simulink model "TST_EISGov_SelectParameter"  (R2016b)
settings: Solver=FixedStepDiscrete  StartTime=0.0  StopTime=simTime  FixedStep=sampleTime  RelTol=1e-3
values from neighbouring files (symbols this model uses):
  testCase = 1    [initTST_EISGov_SelectParameter_001.m]
libraries: simulink x26, UnitTest_Lib x24
(part 3 of 3)

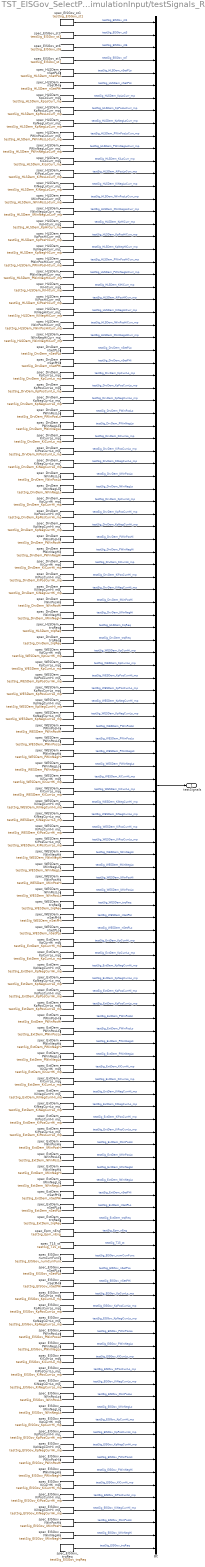
== system TST_EISGov_SelectParameter/simulationInput/testSignals_R001 ==
  BC : BusCreator  Inputs=122
  spec_DrvDem_IWinNegHi : FromWorkspace  VariableName=testSig_DrvDem_IWinNegHi  Interpolate=off  OutputAfterFinalValue=Holding final value
  spec_DrvDem_IWinNegLo : FromWorkspace  VariableName=testSig_DrvDem_IWinNegLo  Interpolate=off  OutputAfterFinalValue=Holding final value
  spec_DrvDem_IWinPosHi : FromWorkspace  VariableName=testSig_DrvDem_IWinPosHi  Interpolate=off  OutputAfterFinalValue=Holding final value
  spec_DrvDem_IWinPosLo : FromWorkspace  VariableName=testSig_DrvDem_IWinPosLo  Interpolate=off  OutputAfterFinalValue=Holding final value
  spec_DrvDem_KiCurrHi_mp : FromWorkspace  VariableName=testSig_DrvDem_KiCurrHi_mp  Interpolate=off  OutputAfterFinalValue=Holding final value
  spec_DrvDem_KiCurrLo_mp : FromWorkspace  VariableName=testSig_DrvDem_KiCurrLo_mp  Interpolate=off  OutputAfterFinalValue=Holding final value
  spec_DrvDem_KiNegCurrHi_mp : FromWorkspace  VariableName=testSig_DrvDem_KiNegCurrHi_mp  Interpolate=off  OutputAfterFinalValue=Holding final value
  spec_DrvDem_KiNegCurrLo_mp : FromWorkspace  VariableName=testSig_DrvDem_KiNegCurrLo_mp  Interpolate=off  OutputAfterFinalValue=Holding final value
  spec_DrvDem_KiPosCurrHi_mp : FromWorkspace  VariableName=testSig_DrvDem_KiPosCurrHi_mp  Interpolate=off  OutputAfterFinalValue=Holding final value
  spec_DrvDem_KiPosCurrLo_mp : FromWorkspace  VariableName=testSig_DrvDem_KiPosCurrLo_mp  Interpolate=off  OutputAfterFinalValue=Holding final value
  spec_DrvDem_KpCurrHi_mp : FromWorkspace  VariableName=testSig_DrvDem_KpCurrHi_mp  Interpolate=off  OutputAfterFinalValue=Holding final value
  spec_DrvDem_KpCurrLo_mp : FromWorkspace  VariableName=testSig_DrvDem_KpCurrLo_mp  Interpolate=off  OutputAfterFinalValue=Holding final value
  spec_DrvDem_KpNegCurrHi_mp : FromWorkspace  VariableName=testSig_DrvDem_KpNegCurrHi_mp  Interpolate=off  OutputAfterFinalValue=Holding final value
  spec_DrvDem_KpNegCurrLo_mp : FromWorkspace  VariableName=testSig_DrvDem_KpNegCurrLo_mp  Interpolate=off  OutputAfterFinalValue=Holding final value
  spec_DrvDem_KpPosCurrHi_mp : FromWorkspace  VariableName=testSig_DrvDem_KpPosCurrHi_mp  Interpolate=off  OutputAfterFinalValue=Holding final value
  spec_DrvDem_KpPosCurrLo_mp : FromWorkspace  VariableName=testSig_DrvDem_KpPosCurrLo_mp  Interpolate=off  OutputAfterFinalValue=Holding final value
  spec_DrvDem_PWinNegHi : FromWorkspace  VariableName=testSig_DrvDem_PWinNegHi  Interpolate=off  OutputAfterFinalValue=Holding final value
  spec_DrvDem_PWinNegLo : FromWorkspace  VariableName=testSig_DrvDem_PWinNegLo  Interpolate=off  OutputAfterFinalValue=Holding final value
  spec_DrvDem_PWinPosHi : FromWorkspace  VariableName=testSig_DrvDem_PWinPosHi  Interpolate=off  OutputAfterFinalValue=Holding final value
  spec_DrvDem_PWinPosLo : FromWorkspace  VariableName=testSig_DrvDem_PWinPosLo  Interpolate=off  OutputAfterFinalValue=Holding final value
  spec_DrvDem_nSetPHi : FromWorkspace  VariableName=testSig_DrvDem_nSetPHi  Interpolate=off  OutputAfterFinalValue=Holding final value
  spec_DrvDem_nSetPLo : FromWorkspace  VariableName=testSig_DrvDem_nSetPLo  Interpolate=off  OutputAfterFinalValue=Holding final value
  spec_DrvDem_trqReq : FromWorkspace  VariableName=testSig_DrvDem_trqReq  Interpolate=off  OutputAfterFinalValue=Holding final value
  spec_EISGov_IWinNegHi : FromWorkspace  VariableName=testSig_EISGov_IWinNegHi  Interpolate=off  OutputAfterFinalValue=Holding final value
  spec_EISGov_IWinNegLo : FromWorkspace  VariableName=testSig_EISGov_IWinNegLo  Interpolate=off  OutputAfterFinalValue=Holding final value
  spec_EISGov_IWinPosHi : FromWorkspace  VariableName=testSig_EISGov_IWinPosHi  Interpolate=off  OutputAfterFinalValue=Holding final value
  spec_EISGov_IWinPosLo : FromWorkspace  VariableName=testSig_EISGov_IWinPosLo  Interpolate=off  OutputAfterFinalValue=Holding final value
  spec_EISGov_KiCurrHi_mp : FromWorkspace  VariableName=testSig_EISGov_KiCurrHi_mp  Interpolate=off  OutputAfterFinalValue=Holding final value
  spec_EISGov_KiCurrLo_mp : FromWorkspace  VariableName=testSig_EISGov_KiCurrLo_mp  Interpolate=off  OutputAfterFinalValue=Holding final value
  spec_EISGov_KiNegCurrHi_mp : FromWorkspace  VariableName=testSig_EISGov_KiNegCurrHi_mp  Interpolate=off  OutputAfterFinalValue=Holding final value
  spec_EISGov_KiNegCurrLo_mp : FromWorkspace  VariableName=testSig_EISGov_KiNegCurrLo_mp  Interpolate=off  OutputAfterFinalValue=Holding final value
  spec_EISGov_KiPosCurrHi_mp : FromWorkspace  VariableName=testSig_EISGov_KiPosCurrHi_mp  Interpolate=off  OutputAfterFinalValue=Holding final value
  spec_EISGov_KiPosCurrLo_mp : FromWorkspace  VariableName=testSig_EISGov_KiPosCurrLo_mp  Interpolate=off  OutputAfterFinalValue=Holding final value
  spec_EISGov_KpCurrHi_mp : FromWorkspace  VariableName=testSig_EISGov_KpCurrHi_mp  Interpolate=off  OutputAfterFinalValue=Holding final value
  spec_EISGov_KpCurrLo_mp : FromWorkspace  VariableName=testSig_EISGov_KpCurrLo_mp  Interpolate=off  OutputAfterFinalValue=Holding final value
  spec_EISGov_KpNegCurrHi_mp : FromWorkspace  VariableName=testSig_EISGov_KpNegCurrHi_mp  Interpolate=off  OutputAfterFinalValue=Holding final value
  spec_EISGov_KpNegCurrLo_mp : FromWorkspace  VariableName=testSig_EISGov_KpNegCurrLo_mp  Interpolate=off  OutputAfterFinalValue=Holding final value
  spec_EISGov_KpPosCurrHi_mp : FromWorkspace  VariableName=testSig_EISGov_KpPosCurrHi_mp  Interpolate=off  OutputAfterFinalValue=Holding final value
  spec_EISGov_KpPosCurrLo_mp : FromWorkspace  VariableName=testSig_EISGov_KpPosCurrLo_mp  Interpolate=off  OutputAfterFinalValue=Holding final value
  spec_EISGov_PWinNegHi : FromWorkspace  VariableName=testSig_EISGov_PWinNegHi  Interpolate=off  OutputAfterFinalValue=Holding final value
  spec_EISGov_PWinNegLo : FromWorkspace  VariableName=testSig_EISGov_PWinNegLo  Interpolate=off  OutputAfterFinalValue=Holding final value
  spec_EISGov_PWinPosHi : FromWorkspace  VariableName=testSig_EISGov_PWinPosHi  Interpolate=off  OutputAfterFinalValue=Holding final value
  spec_EISGov_PWinPosLo : FromWorkspace  VariableName=testSig_EISGov_PWinPosLo  Interpolate=off  OutputAfterFinalValue=Holding final value
  spec_EISGov_nSetPHi : FromWorkspace  VariableName=testSig_EISGov_nSetPHi  Interpolate=off  OutputAfterFinalValue=Holding final value
  spec_EISGov_nSetPLo : FromWorkspace  VariableName=testSig_EISGov_nSetPLo  Interpolate=off  OutputAfterFinalValue=Holding final value
  spec_EISGov_numCurrFunc : FromWorkspace  VariableName=testSig_EISGov_numCurrFunc  Interpolate=off  OutputAfterFinalValue=Holding final value
  spec_EISGov_st1 : FromWorkspace  VariableName=testSig_EISGov_st1  Interpolate=off  OutputAfterFinalValue=Holding final value
  spec_EISGov_st3 : FromWorkspace  VariableName=testSig_EISGov_st3  Interpolate=off  OutputAfterFinalValue=Holding final value
  spec_EISGov_st6 : FromWorkspace  VariableName=testSig_EISGov_st6  Interpolate=off  OutputAfterFinalValue=Holding final value
  spec_EISGov_st7 : FromWorkspace  VariableName=testSig_EISGov_st7  Interpolate=off  OutputAfterFinalValue=Holding final value
  spec_EISGov_trqReq : FromWorkspace  VariableName=testSig_EISGov_trqReq  Interpolate=off  OutputAfterFinalValue=Holding final value
  spec_Epm_nEng : FromWorkspace  VariableName=testSig_Epm_nEng  Interpolate=off  OutputAfterFinalValue=Holding final value
  spec_ExtDem_IWinNegHi : FromWorkspace  VariableName=testSig_ExtDem_IWinNegHi  Interpolate=off  OutputAfterFinalValue=Holding final value
  spec_ExtDem_IWinNegLo : FromWorkspace  VariableName=testSig_ExtDem_IWinNegLo  Interpolate=off  OutputAfterFinalValue=Holding final value
  spec_ExtDem_IWinPosHi : FromWorkspace  VariableName=testSig_ExtDem_IWinPosHi  Interpolate=off  OutputAfterFinalValue=Holding final value
  spec_ExtDem_IWinPosLo : FromWorkspace  VariableName=testSig_ExtDem_IWinPosLo  Interpolate=off  OutputAfterFinalValue=Holding final value
  spec_ExtDem_KiCurrHi_mp : FromWorkspace  VariableName=testSig_ExtDem_KiCurrHi_mp  Interpolate=off  OutputAfterFinalValue=Holding final value
  spec_ExtDem_KiCurrLo_mp : FromWorkspace  VariableName=testSig_ExtDem_KiCurrLo_mp  Interpolate=off  OutputAfterFinalValue=Holding final value
  spec_ExtDem_KiNegCurrHi_mp : FromWorkspace  VariableName=testSig_ExtDem_KiNegCurrHi_mp  Interpolate=off  OutputAfterFinalValue=Holding final value
  spec_ExtDem_KiNegCurrLo_mp : FromWorkspace  VariableName=testSig_ExtDem_KiNegCurrLo_mp  Interpolate=off  OutputAfterFinalValue=Holding final value
  spec_ExtDem_KiPosCurrHi_mp : FromWorkspace  VariableName=testSig_ExtDem_KiPosCurrHi_mp  Interpolate=off  OutputAfterFinalValue=Holding final value
  spec_ExtDem_KiPosCurrLo_mp : FromWorkspace  VariableName=testSig_ExtDem_KiPosCurrLo_mp  Interpolate=off  OutputAfterFinalValue=Holding final value
  spec_ExtDem_KpCurrHi_mp : FromWorkspace  VariableName=testSig_ExtDem_KpCurrHi_mp  Interpolate=off  OutputAfterFinalValue=Holding final value
  spec_ExtDem_KpCurrLo_mp : FromWorkspace  VariableName=testSig_ExtDem_KpCurrLo_mp  Interpolate=off  OutputAfterFinalValue=Holding final value
  spec_ExtDem_KpNegCurrHi_mp : FromWorkspace  VariableName=testSig_ExtDem_KpNegCurrHi_mp  Interpolate=off  OutputAfterFinalValue=Holding final value
  spec_ExtDem_KpNegCurrLo_mp : FromWorkspace  VariableName=testSig_ExtDem_KpNegCurrLo_mp  Interpolate=off  OutputAfterFinalValue=Holding final value
  spec_ExtDem_KpPosCurrHi_mp : FromWorkspace  VariableName=testSig_ExtDem_KpPosCurrHi_mp  Interpolate=off  OutputAfterFinalValue=Holding final value
  spec_ExtDem_KpPosCurrLo_mp : FromWorkspace  VariableName=testSig_ExtDem_KpPosCurrLo_mp  Interpolate=off  OutputAfterFinalValue=Holding final value
  spec_ExtDem_PWinNegHi : FromWorkspace  VariableName=testSig_ExtDem_PWinNegHi  Interpolate=off  OutputAfterFinalValue=Holding final value
  spec_ExtDem_PWinNegLo : FromWorkspace  VariableName=testSig_ExtDem_PWinNegLo  Interpolate=off  OutputAfterFinalValue=Holding final value
  spec_ExtDem_PWinPosHi : FromWorkspace  VariableName=testSig_ExtDem_PWinPosHi  Interpolate=off  OutputAfterFinalValue=Holding final value
  spec_ExtDem_PWinPosLo : FromWorkspace  VariableName=testSig_ExtDem_PWinPosLo  Interpolate=off  OutputAfterFinalValue=Holding final value
  spec_ExtDem_nSetPHi : FromWorkspace  VariableName=testSig_ExtDem_nSetPHi  Interpolate=off  OutputAfterFinalValue=Holding final value
  spec_ExtDem_nSetPLo : FromWorkspace  VariableName=testSig_ExtDem_nSetPLo  Interpolate=off  OutputAfterFinalValue=Holding final value
  spec_ExtDem_trqReq : FromWorkspace  VariableName=testSig_ExtDem_trqReq  Interpolate=off  OutputAfterFinalValue=Holding final value
  spec_HLSDem_IWinNegHiCurr_mp : FromWorkspace  VariableName=testSig_HLSDem_IWinNegHiCurr_mp  Interpolate=off  OutputAfterFinalValue=Holding final value
  spec_HLSDem_IWinNegLoCurr_mp : FromWorkspace  VariableName=testSig_HLSDem_IWinNegLoCurr_mp  Interpolate=off  OutputAfterFinalValue=Holding final value
  spec_HLSDem_IWinPosHiCurr_mp : FromWorkspace  VariableName=testSig_HLSDem_IWinPosHiCurr_mp  Interpolate=off  OutputAfterFinalValue=Holding final value
  spec_HLSDem_IWinPosLoCurr_mp : FromWorkspace  VariableName=testSig_HLSDem_IWinPosLoCurr_mp  Interpolate=off  OutputAfterFinalValue=Holding final value
  spec_HLSDem_KiHiCurr_mp : FromWorkspace  VariableName=testSig_HLSDem_KiHiCurr_mp  Interpolate=off  OutputAfterFinalValue=Holding final value
  spec_HLSDem_KiLoCurr_mp : FromWorkspace  VariableName=testSig_HLSDem_KiLoCurr_mp  Interpolate=off  OutputAfterFinalValue=Holding final value
  spec_HLSDem_KiNegHiCurr_mp : FromWorkspace  VariableName=testSig_HLSDem_KiNegHiCurr_mp  Interpolate=off  OutputAfterFinalValue=Holding final value
  spec_HLSDem_KiNegLoCurr_mp : FromWorkspace  VariableName=testSig_HLSDem_KiNegLoCurr_mp  Interpolate=off  OutputAfterFinalValue=Holding final value
  spec_HLSDem_KiPosHiCurr_mp : FromWorkspace  VariableName=testSig_HLSDem_KiPosHiCurr_mp  Interpolate=off  OutputAfterFinalValue=Holding final value
  spec_HLSDem_KiPosLoCurr_mp : FromWorkspace  VariableName=testSig_HLSDem_KiPosLoCurr_mp  Interpolate=off  OutputAfterFinalValue=Holding final value
  spec_HLSDem_KpHiCurr_mp : FromWorkspace  VariableName=testSig_HLSDem_KpHiCurr_mp  Interpolate=off  OutputAfterFinalValue=Holding final value
  spec_HLSDem_KpLoCurr_mp : FromWorkspace  VariableName=testSig_HLSDem_KpLoCurr_mp  Interpolate=off  OutputAfterFinalValue=Holding final value
  spec_HLSDem_KpNegHiCurr_mp : FromWorkspace  VariableName=testSig_HLSDem_KpNegHiCurr_mp  Interpolate=off  OutputAfterFinalValue=Holding final value
  spec_HLSDem_KpNegLoCurr_mp : FromWorkspace  VariableName=testSig_HLSDem_KpNegLoCurr_mp  Interpolate=off  OutputAfterFinalValue=Holding final value
  spec_HLSDem_KpPosHiCurr_mp : FromWorkspace  VariableName=testSig_HLSDem_KpPosHiCurr_mp  Interpolate=off  OutputAfterFinalValue=Holding final value
  spec_HLSDem_KpPosLoCurr_mp : FromWorkspace  VariableName=testSig_HLSDem_KpPosLoCurr_mp  Interpolate=off  OutputAfterFinalValue=Holding final value
  spec_HLSDem_PWinNegHiCurr_mp : FromWorkspace  VariableName=testSig_HLSDem_PWinNegHiCurr_mp  Interpolate=off  OutputAfterFinalValue=Holding final value
  spec_HLSDem_PWinNegLoCurr_mp : FromWorkspace  VariableName=testSig_HLSDem_PWinNegLoCurr_mp  Interpolate=off  OutputAfterFinalValue=Holding final value
  spec_HLSDem_PWinPosHiCurr_mp : FromWorkspace  VariableName=testSig_HLSDem_PWinPosHiCurr_mp  Interpolate=off  OutputAfterFinalValue=Holding final value
  spec_HLSDem_PWinPosLoCurr_mp : FromWorkspace  VariableName=testSig_HLSDem_PWinPosLoCurr_mp  Interpolate=off  OutputAfterFinalValue=Holding final value
  spec_HLSDem_nSetPHi : FromWorkspace  VariableName=testSig_HLSDem_nSetPHi  Interpolate=off  OutputAfterFinalValue=Holding final value
  spec_HLSDem_nSetPLo : FromWorkspace  VariableName=testSig_HLSDem_nSetPLo  Interpolate=off  OutputAfterFinalValue=Holding final value
  spec_HLSDem_trqReq : FromWorkspace  VariableName=testSig_HLSDem_trqReq  Interpolate=off  OutputAfterFinalValue=Holding final value
  spec_T15_st : FromWorkspace  VariableName=testSig_T15_st  Interpolate=off  OutputAfterFinalValue=Holding final value
  spec_WESDem_IWinNegHi : FromWorkspace  VariableName=testSig_WESDem_IWinNegHi  Interpolate=off  OutputAfterFinalValue=Holding final value
  spec_WESDem_IWinNegLo : FromWorkspace  VariableName=testSig_WESDem_IWinNegLo  Interpolate=off  OutputAfterFinalValue=Holding final value
  spec_WESDem_IWinPosHi : FromWorkspace  VariableName=testSig_WESDem_IWinPosHi  Interpolate=off  OutputAfterFinalValue=Holding final value
  spec_WESDem_IWinPosLo : FromWorkspace  VariableName=testSig_WESDem_IWinPosLo  Interpolate=off  OutputAfterFinalValue=Holding final value
  spec_WESDem_KiCurrHi_mp : FromWorkspace  VariableName=testSig_WESDem_KiCurrHi_mp  Interpolate=off  OutputAfterFinalValue=Holding final value
  spec_WESDem_KiCurrLo_mp : FromWorkspace  VariableName=testSig_WESDem_KiCurrLo_mp  Interpolate=off  OutputAfterFinalValue=Holding final value
  spec_WESDem_KiNegCurrHi_mp : FromWorkspace  VariableName=testSig_WESDem_KiNegCurrHi_mp  Interpolate=off  OutputAfterFinalValue=Holding final value
  spec_WESDem_KiNegCurrLo_mp : FromWorkspace  VariableName=testSig_WESDem_KiNegCurrLo_mp  Interpolate=off  OutputAfterFinalValue=Holding final value
  spec_WESDem_KiPosCurrHi_mp : FromWorkspace  VariableName=testSig_WESDem_KiPosCurrHi_mp  Interpolate=off  OutputAfterFinalValue=Holding final value
  spec_WESDem_KiPosCurrLo_mp : FromWorkspace  VariableName=testSig_WESDem_KiPosCurrLo_mp  Interpolate=off  OutputAfterFinalValue=Holding final value
  spec_WESDem_KpCurrHi_mp : FromWorkspace  VariableName=testSig_WESDem_KpCurrHi_mp  Interpolate=off  OutputAfterFinalValue=Holding final value
  spec_WESDem_KpCurrLo_mp : FromWorkspace  VariableName=testSig_WESDem_KpCurrLo_mp  Interpolate=off  OutputAfterFinalValue=Holding final value
  spec_WESDem_KpNegCurrHi_mp : FromWorkspace  VariableName=testSig_WESDem_KpNegCurrHi_mp  Interpolate=off  OutputAfterFinalValue=Holding final value
  spec_WESDem_KpNegCurrLo_mp : FromWorkspace  VariableName=testSig_WESDem_KpNegCurrLo_mp  Interpolate=off  OutputAfterFinalValue=Holding final value
  spec_WESDem_KpPosCurrHi_mp : FromWorkspace  VariableName=testSig_WESDem_KpPosCurrHi_mp  Interpolate=off  OutputAfterFinalValue=Holding final value
  spec_WESDem_KpPosCurrLo_mp : FromWorkspace  VariableName=testSig_WESDem_KpPosCurrLo_mp  Interpolate=off  OutputAfterFinalValue=Holding final value
  spec_WESDem_PWinNegHi : FromWorkspace  VariableName=testSig_WESDem_PWinNegHi  Interpolate=off  OutputAfterFinalValue=Holding final value
  spec_WESDem_PWinNegLo : FromWorkspace  VariableName=testSig_WESDem_PWinNegLo  Interpolate=off  OutputAfterFinalValue=Holding final value
  spec_WESDem_PWinPosHi : FromWorkspace  VariableName=testSig_WESDem_PWinPosHi  Interpolate=off  OutputAfterFinalValue=Holding final value
  spec_WESDem_PWinPosLo : FromWorkspace  VariableName=testSig_WESDem_PWinPosLo  Interpolate=off  OutputAfterFinalValue=Holding final value
  spec_WESDem_nSetPHi : FromWorkspace  VariableName=testSig_WESDem_nSetPHi  Interpolate=off  OutputAfterFinalValue=Holding final value
  spec_WESDem_nSetPLo : FromWorkspace  VariableName=testSig_WESDem_nSetPLo  Interpolate=off  OutputAfterFinalValue=Holding final value
  spec_WESDem_trqReq : FromWorkspace  VariableName=testSig_WESDem_trqReq  Interpolate=off  OutputAfterFinalValue=Holding final value
  testSignals : Outport
  wires:
  BC/1 -> testSignals/1
  spec_EISGov_st1/1 -> BC/1  "testSig_EISGov_st1"
  spec_EISGov_st3/1 -> BC/2  "testSig_EISGov_st3"
  spec_EISGov_st6/1 -> BC/3  "testSig_EISGov_st6"
  spec_EISGov_st7/1 -> BC/4  "testSig_EISGov_st7"
  spec_HLSDem_nSetPLo/1 -> BC/5  "testSig_HLSDem_nSetPLo"
  spec_HLSDem_nSetPHi/1 -> BC/6  "testSig_HLSDem_nSetPHi"
  spec_HLSDem_KpLoCurr_mp/1 -> BC/7  "testSig_HLSDem_KpLoCurr_mp"
  spec_HLSDem_KpPosLoCurr_mp/1 -> BC/8  "testSig_HLSDem_KpPosLoCurr_mp"
  spec_HLSDem_KpNegLoCurr_mp/1 -> BC/9  "testSig_HLSDem_KpNegLoCurr_mp"
  spec_HLSDem_PWinPosLoCurr_mp/1 -> BC/10  "testSig_HLSDem_PWinPosLoCurr_mp"
  spec_HLSDem_PWinNegLoCurr_mp/1 -> BC/11  "testSig_HLSDem_PWinNegLoCurr_mp"
  spec_HLSDem_KiLoCurr_mp/1 -> BC/12  "testSig_HLSDem_KiLoCurr_mp"
  spec_HLSDem_KiPosLoCurr_mp/1 -> BC/13  "testSig_HLSDem_KiPosLoCurr_mp"
  spec_HLSDem_KiNegLoCurr_mp/1 -> BC/14  "testSig_HLSDem_KiNegLoCurr_mp"
  spec_HLSDem_IWinPosLoCurr_mp/1 -> BC/15  "testSig_HLSDem_IWinPosLoCurr_mp"
  spec_HLSDem_IWinNegLoCurr_mp/1 -> BC/16  "testSig_HLSDem_IWinNegLoCurr_mp"
  spec_HLSDem_KpHiCurr_mp/1 -> BC/17  "testSig_HLSDem_KpHiCurr_mp"
  spec_HLSDem_KpPosHiCurr_mp/1 -> BC/18  "testSig_HLSDem_KpPosHiCurr_mp"
  spec_HLSDem_KpNegHiCurr_mp/1 -> BC/19  "testSig_HLSDem_KpNegHiCurr_mp"
  spec_HLSDem_PWinPosHiCurr_mp/1 -> BC/20  "testSig_HLSDem_PWinPosHiCurr_mp"
  spec_HLSDem_PWinNegHiCurr_mp/1 -> BC/21  "testSig_HLSDem_PWinNegHiCurr_mp"
  spec_HLSDem_KiHiCurr_mp/1 -> BC/22  "testSig_HLSDem_KiHiCurr_mp"
  spec_HLSDem_KiPosHiCurr_mp/1 -> BC/23  "testSig_HLSDem_KiPosHiCurr_mp"
  spec_HLSDem_KiNegHiCurr_mp/1 -> BC/24  "testSig_HLSDem_KiNegHiCurr_mp"
  spec_HLSDem_IWinPosHiCurr_mp/1 -> BC/25  "testSig_HLSDem_IWinPosHiCurr_mp"
  spec_HLSDem_IWinNegHiCurr_mp/1 -> BC/26  "testSig_HLSDem_IWinNegHiCurr_mp"
  spec_DrvDem_nSetPLo/1 -> BC/27  "testSig_DrvDem_nSetPLo"
  spec_DrvDem_nSetPHi/1 -> BC/28  "testSig_DrvDem_nSetPHi"
  spec_DrvDem_KpCurrLo_mp/1 -> BC/29  "testSig_DrvDem_KpCurrLo_mp"
  spec_DrvDem_KpPosCurrLo_mp/1 -> BC/30  "testSig_DrvDem_KpPosCurrLo_mp"
  spec_DrvDem_KpNegCurrLo_mp/1 -> BC/31  "testSig_DrvDem_KpNegCurrLo_mp"
  spec_DrvDem_PWinPosLo/1 -> BC/32  "testSig_DrvDem_PWinPosLo"
  spec_DrvDem_PWinNegLo/1 -> BC/33  "testSig_DrvDem_PWinNegLo"
  spec_DrvDem_KiCurrLo_mp/1 -> BC/34  "testSig_DrvDem_KiCurrLo_mp"
  spec_DrvDem_KiPosCurrLo_mp/1 -> BC/35  "testSig_DrvDem_KiPosCurrLo_mp"
  spec_DrvDem_KiNegCurrLo_mp/1 -> BC/36  "testSig_DrvDem_KiNegCurrLo_mp"
  spec_DrvDem_IWinPosLo/1 -> BC/37  "testSig_DrvDem_IWinPosLo"
  spec_DrvDem_IWinNegLo/1 -> BC/38  "testSig_DrvDem_IWinNegLo"
  spec_DrvDem_KpCurrHi_mp/1 -> BC/39  "testSig_DrvDem_KpCurrHi_mp"
  spec_DrvDem_KpPosCurrHi_mp/1 -> BC/40  "testSig_DrvDem_KpPosCurrHi_mp"
  spec_DrvDem_KpNegCurrHi_mp/1 -> BC/41  "testSig_DrvDem_KpNegCurrHi_mp"
  spec_DrvDem_PWinPosHi/1 -> BC/42  "testSig_DrvDem_PWinPosHi"
  spec_DrvDem_PWinNegHi/1 -> BC/43  "testSig_DrvDem_PWinNegHi"
  spec_DrvDem_KiCurrHi_mp/1 -> BC/44  "testSig_DrvDem_KiCurrHi_mp"
  spec_DrvDem_KiPosCurrHi_mp/1 -> BC/45  "testSig_DrvDem_KiPosCurrHi_mp"
  spec_DrvDem_KiNegCurrHi_mp/1 -> BC/46  "testSig_DrvDem_KiNegCurrHi_mp"
  spec_DrvDem_IWinPosHi/1 -> BC/47  "testSig_DrvDem_IWinPosHi"
  spec_DrvDem_IWinNegHi/1 -> BC/48  "testSig_DrvDem_IWinNegHi"
  spec_HLSDem_trqReq/1 -> BC/49  "testSig_HLSDem_trqReq"
  spec_DrvDem_trqReq/1 -> BC/50  "testSig_DrvDem_trqReq"
  spec_WESDem_KpCurrHi_mp/1 -> BC/51  "testSig_WESDem_KpCurrHi_mp"
  spec_WESDem_KpCurrLo_mp/1 -> BC/52  "testSig_WESDem_KpCurrLo_mp"
  spec_WESDem_KpPosCurrHi_mp/1 -> BC/53  "testSig_WESDem_KpPosCurrHi_mp"
  spec_WESDem_KpPosCurrLo_mp/1 -> BC/54  "testSig_WESDem_KpPosCurrLo_mp"
  spec_WESDem_KpNegCurrHi_mp/1 -> BC/55  "testSig_WESDem_KpNegCurrHi_mp"
  spec_WESDem_KpNegCurrLo_mp/1 -> BC/56  "testSig_WESDem_KpNegCurrLo_mp"
  spec_WESDem_PWinPosHi/1 -> BC/57  "testSig_WESDem_PWinPosHi"
  spec_WESDem_PWinPosLo/1 -> BC/58  "testSig_WESDem_PWinPosLo"
  spec_WESDem_PWinNegHi/1 -> BC/59  "testSig_WESDem_PWinNegHi"
  spec_WESDem_PWinNegLo/1 -> BC/60  "testSig_WESDem_PWinNegLo"
  spec_WESDem_KiCurrHi_mp/1 -> BC/61  "testSig_WESDem_KiCurrHi_mp"
  spec_WESDem_KiCurrLo_mp/1 -> BC/62  "testSig_WESDem_KiCurrLo_mp"
  spec_WESDem_KiNegCurrHi_mp/1 -> BC/63  "testSig_WESDem_KiNegCurrHi_mp"
  spec_WESDem_KiNegCurrLo_mp/1 -> BC/64  "testSig_WESDem_KiNegCurrLo_mp"
  spec_WESDem_KiPosCurrHi_mp/1 -> BC/65  "testSig_WESDem_KiPosCurrHi_mp"
  spec_WESDem_KiPosCurrLo_mp/1 -> BC/66  "testSig_WESDem_KiPosCurrLo_mp"
  spec_WESDem_IWinNegHi/1 -> BC/67  "testSig_WESDem_IWinNegHi"
  spec_WESDem_IWinNegLo/1 -> BC/68  "testSig_WESDem_IWinNegLo"
  spec_WESDem_IWinPosHi/1 -> BC/69  "testSig_WESDem_IWinPosHi"
  spec_WESDem_IWinPosLo/1 -> BC/70  "testSig_WESDem_IWinPosLo"
  spec_WESDem_trqReq/1 -> BC/71  "testSig_WESDem_trqReq"
  spec_WESDem_nSetPHi/1 -> BC/72  "testSig_WESDem_nSetPHi"
  spec_WESDem_nSetPLo/1 -> BC/73  "testSig_WESDem_nSetPLo"
  spec_ExtDem_KpCurrHi_mp/1 -> BC/74  "testSig_ExtDem_KpCurrHi_mp"
  spec_ExtDem_KpCurrLo_mp/1 -> BC/75  "testSig_ExtDem_KpCurrLo_mp"
  spec_ExtDem_KpNegCurrHi_mp/1 -> BC/76  "testSig_ExtDem_KpNegCurrHi_mp"
  spec_ExtDem_KpNegCurrLo_mp/1 -> BC/77  "testSig_ExtDem_KpNegCurrLo_mp"
  spec_ExtDem_KpPosCurrHi_mp/1 -> BC/78  "testSig_ExtDem_KpPosCurrHi_mp"
  spec_ExtDem_KpPosCurrLo_mp/1 -> BC/79  "testSig_ExtDem_KpPosCurrLo_mp"
  spec_ExtDem_PWinPosHi/1 -> BC/80  "testSig_ExtDem_PWinPosHi"
  spec_ExtDem_PWinPosLo/1 -> BC/81  "testSig_ExtDem_PWinPosLo"
  spec_ExtDem_PWinNegHi/1 -> BC/82  "testSig_ExtDem_PWinNegHi"
  spec_ExtDem_PWinNegLo/1 -> BC/83  "testSig_ExtDem_PWinNegLo"
  spec_ExtDem_KiCurrHi_mp/1 -> BC/84  "testSig_ExtDem_KiCurrHi_mp"
  spec_ExtDem_KiCurrLo_mp/1 -> BC/85  "testSig_ExtDem_KiCurrLo_mp"
  spec_ExtDem_KiNegCurrHi_mp/1 -> BC/86  "testSig_ExtDem_KiNegCurrHi_mp"
  spec_ExtDem_KiNegCurrLo_mp/1 -> BC/87  "testSig_ExtDem_KiNegCurrLo_mp"
  spec_ExtDem_KiPosCurrHi_mp/1 -> BC/88  "testSig_ExtDem_KiPosCurrHi_mp"
  spec_ExtDem_KiPosCurrLo_mp/1 -> BC/89  "testSig_ExtDem_KiPosCurrLo_mp"
  spec_ExtDem_IWinPosHi/1 -> BC/90  "testSig_ExtDem_IWinPosHi"
  spec_ExtDem_IWinPosLo/1 -> BC/91  "testSig_ExtDem_IWinPosLo"
  spec_ExtDem_IWinNegHi/1 -> BC/92  "testSig_ExtDem_IWinNegHi"
  spec_ExtDem_IWinNegLo/1 -> BC/93  "testSig_ExtDem_IWinNegLo"
  spec_ExtDem_nSetPHi/1 -> BC/94  "testSig_ExtDem_nSetPHi"
  spec_ExtDem_nSetPLo/1 -> BC/95  "testSig_ExtDem_nSetPLo"
  spec_ExtDem_trqReq/1 -> BC/96  "testSig_ExtDem_trqReq"
  spec_Epm_nEng/1 -> BC/97  "testSig_Epm_nEng"
  spec_T15_st/1 -> BC/98  "testSig_T15_st"
  spec_EISGov_numCurrFunc/1 -> BC/99  "testSig_EISGov_numCurrFunc"
  spec_EISGov_nSetPLo/1 -> BC/100  "testSig_EISGov_nSetPLo"
  spec_EISGov_nSetPHi/1 -> BC/101  "testSig_EISGov_nSetPHi"
  spec_EISGov_KpCurrLo_mp/1 -> BC/102  "testSig_EISGov_KpCurrLo_mp"
  spec_EISGov_KpPosCurrLo_mp/1 -> BC/103  "testSig_EISGov_KpPosCurrLo_mp"
  spec_EISGov_KpNegCurrLo_mp/1 -> BC/104  "testSig_EISGov_KpNegCurrLo_mp"
  spec_EISGov_PWinPosLo/1 -> BC/105  "testSig_EISGov_PWinPosLo"
  spec_EISGov_PWinNegLo/1 -> BC/106  "testSig_EISGov_PWinNegLo"
  spec_EISGov_KiCurrLo_mp/1 -> BC/107  "testSig_EISGov_KiCurrLo_mp"
  spec_EISGov_KiPosCurrLo_mp/1 -> BC/108  "testSig_EISGov_KiPosCurrLo_mp"
  spec_EISGov_KiNegCurrLo_mp/1 -> BC/109  "testSig_EISGov_KiNegCurrLo_mp"
  spec_EISGov_IWinPosLo/1 -> BC/110  "testSig_EISGov_IWinPosLo"
  spec_EISGov_IWinNegLo/1 -> BC/111  "testSig_EISGov_IWinNegLo"
  spec_EISGov_KpCurrHi_mp/1 -> BC/112  "testSig_EISGov_KpCurrHi_mp"
  spec_EISGov_KpPosCurrHi_mp/1 -> BC/113  "testSig_EISGov_KpPosCurrHi_mp"
  spec_EISGov_KpNegCurrHi_mp/1 -> BC/114  "testSig_EISGov_KpNegCurrHi_mp"
  spec_EISGov_PWinPosHi/1 -> BC/115  "testSig_EISGov_PWinPosHi"
  spec_EISGov_PWinNegHi/1 -> BC/116  "testSig_EISGov_PWinNegHi"
  spec_EISGov_KiCurrHi_mp/1 -> BC/117  "testSig_EISGov_KiCurrHi_mp"
  spec_EISGov_KiPosCurrHi_mp/1 -> BC/118  "testSig_EISGov_KiPosCurrHi_mp"
  spec_EISGov_KiNegCurrHi_mp/1 -> BC/119  "testSig_EISGov_KiNegCurrHi_mp"
  spec_EISGov_IWinPosHi/1 -> BC/120  "testSig_EISGov_IWinPosHi"
  spec_EISGov_IWinNegHi/1 -> BC/121  "testSig_EISGov_IWinNegHi"
  spec_EISGov_trqReq/1 -> BC/122  "testSig_EISGov_trqReq"

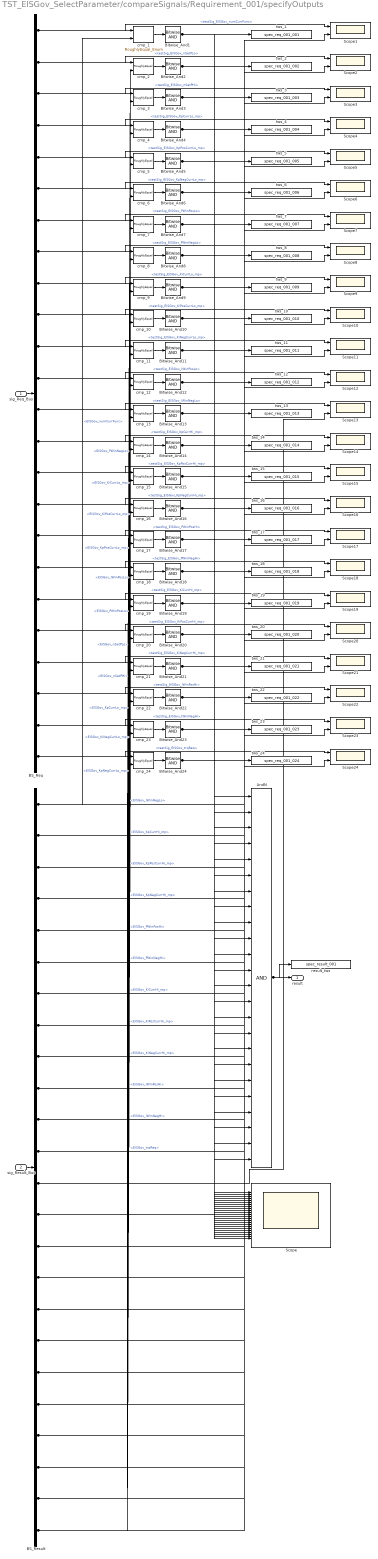
== system TST_EISGov_SelectParameter/compareSignals/Requirement_001/specifyOutputs ==
  sig_Req_Bus : Inport
  sig_Result_Bus : Inport  Port=2
  AndN : Logic  Inputs=24
  BS_Req : BusSelector  OutputSignals=testSig_EISGov_numCurrFunc,testSig_EISGov_nSetPLo,testSig_EISGov_nSetPHi,testSig_EISGov_KpCurrLo_mp,testSig_EISGov_KpPosCurrLo_mp,testSig_EISGov_KpNegCurrLo_mp,testSig_EISGov_PWinPosLo,testSig_EISGov_PWinNegLo,testSig_EISGov_KiCurrLo_mp,testSig_EISGov_KiPosCurrLo_mp,testSig_EISGov_KiNegCurrLo_mp,testSig_EISGov_IWinPosLo,testSig_EISGov_IWinNegLo,testSig_EISGov_KpCurrHi_mp,testSig_EISGov_KpPosCurrHi_mp,testSig_EISGov_KpNegCurrHi_mp,testSig_EISGov_PWinPosHi,testSig_EISGov_PWinNegHi,testSig_EISGov_KiCurrHi_mp,testSig_EISGov_KiPosCurrHi_mp,testSig_EISGov_KiNegCurrHi_mp,testSig_EISGov_IWinPosHi,testSig_EISGov_IWinNegHi,testSig_EISGov_trqReq
  BS_Result : BusSelector  OutputSignals=EISGov_numCurrFunc,EISGov_nSetPLo,EISGov_nSetPHi,EISGov_KpCurrLo_mp,EISGov_KpPosCurrLo_mp,EISGov_KpNegCurrLo_mp,EISGov_PWinPosLo,EISGov_PWinNegLo,EISGov_KiCurrLo_mp,EISGov_KiPosCurrLo_mp,EISGov_KiNegCurrLo_mp,EISGov_IWinPosLo,EISGov_IWinNegLo,EISGov_KpCurrHi_mp,EISGov_KpPosCurrHi_mp,EISGov_KpNegCurrHi_mp,EISGov_PWinPosHi,EISGov_PWinNegHi,EISGov_KiCurrHi_mp,EISGov_KiPosCurrHi_mp,EISGov_KiNegCurrHi_mp,EISGov_IWinPosHi,EISGov_IWinNegHi,EISGov_trqReq
  Bitwise_And{1..24} (24 alike) : simulink/Logic and Bit Operations/Bitwise Operator  logicop=AND  UseBitMask=off  BitMask=bin2dec('11011001')  BitMaskRealWorld=Stored Integer
  Scope : Scope  NumInputPorts=24
  Scope{1..24} (24 alike) : Scope  NumInputPorts=2
  cmp_1 : UnitTest_Lib/RoughlyEqual_Enum  slope=0.1
  cmp_{2..24} (23 alike) : UnitTest_Lib/RoughlyEqual  slope=0.1
  result_tws : ToWorkspace  VariableName=spec_result_001
  tws_1 : ToWorkspace  VariableName=spec_req_001_001
  tws_10 : ToWorkspace  VariableName=spec_req_001_010
  tws_11 : ToWorkspace  VariableName=spec_req_001_011
  tws_12 : ToWorkspace  VariableName=spec_req_001_012
  tws_13 : ToWorkspace  VariableName=spec_req_001_013
  tws_14 : ToWorkspace  VariableName=spec_req_001_014
  tws_15 : ToWorkspace  VariableName=spec_req_001_015
  tws_16 : ToWorkspace  VariableName=spec_req_001_016
  tws_17 : ToWorkspace  VariableName=spec_req_001_017
  tws_18 : ToWorkspace  VariableName=spec_req_001_018
  tws_19 : ToWorkspace  VariableName=spec_req_001_019
  tws_2 : ToWorkspace  VariableName=spec_req_001_002
  tws_20 : ToWorkspace  VariableName=spec_req_001_020
  tws_21 : ToWorkspace  VariableName=spec_req_001_021
  tws_22 : ToWorkspace  VariableName=spec_req_001_022
  tws_23 : ToWorkspace  VariableName=spec_req_001_023
  tws_24 : ToWorkspace  VariableName=spec_req_001_024
  tws_3 : ToWorkspace  VariableName=spec_req_001_003
  tws_4 : ToWorkspace  VariableName=spec_req_001_004
  tws_5 : ToWorkspace  VariableName=spec_req_001_005
  tws_6 : ToWorkspace  VariableName=spec_req_001_006
  tws_7 : ToWorkspace  VariableName=spec_req_001_007
  tws_8 : ToWorkspace  VariableName=spec_req_001_008
  tws_9 : ToWorkspace  VariableName=spec_req_001_009
  result : Outport
  wires:
  sig_Req_Bus/1 -> BS_Req/1
  sig_Result_Bus/1 -> BS_Result/1
  AndN/1 -> result/1, result_tws/1
  BS_Req/1 -> cmp_1/1, Scope1/1  "<testSig_EISGov_numCurrFunc>"
  BS_Result/1 -> cmp_1/2, Scope1/2  "<EISGov_numCurrFunc>"
  cmp_1/1 -> Bitwise_And1/1
  Bitwise_And1/1 -> tws_1/1, AndN/1, Scope/1
  BS_Req/2 -> cmp_2/1, Scope2/1  "<testSig_EISGov_nSetPLo>"
  BS_Result/2 -> cmp_2/2, Scope2/2  "<EISGov_nSetPLo>"
  cmp_2/1 -> Bitwise_And2/1
  Bitwise_And2/1 -> tws_2/1, AndN/2, Scope/2
  BS_Req/3 -> cmp_3/1, Scope3/1  "<testSig_EISGov_nSetPHi>"
  BS_Result/3 -> cmp_3/2, Scope3/2  "<EISGov_nSetPHi>"
  cmp_3/1 -> Bitwise_And3/1
  Bitwise_And3/1 -> tws_3/1, AndN/3, Scope/3
  BS_Req/4 -> cmp_4/1, Scope4/1  "<testSig_EISGov_KpCurrLo_mp>"
  BS_Result/4 -> cmp_4/2, Scope4/2  "<EISGov_KpCurrLo_mp>"
  cmp_4/1 -> Bitwise_And4/1
  Bitwise_And4/1 -> tws_4/1, AndN/4, Scope/4
  BS_Req/5 -> cmp_5/1, Scope5/1  "<testSig_EISGov_KpPosCurrLo_mp>"
  BS_Result/5 -> cmp_5/2, Scope5/2  "<EISGov_KpPosCurrLo_mp>"
  cmp_5/1 -> Bitwise_And5/1
  Bitwise_And5/1 -> tws_5/1, AndN/5, Scope/5
  BS_Req/6 -> cmp_6/1, Scope6/1  "<testSig_EISGov_KpNegCurrLo_mp>"
  BS_Result/6 -> cmp_6/2, Scope6/2  "<EISGov_KpNegCurrLo_mp>"
  cmp_6/1 -> Bitwise_And6/1
  Bitwise_And6/1 -> tws_6/1, AndN/6, Scope/6
  BS_Req/7 -> cmp_7/1, Scope7/1  "<testSig_EISGov_PWinPosLo>"
  BS_Result/7 -> cmp_7/2, Scope7/2  "<EISGov_PWinPosLo>"
  cmp_7/1 -> Bitwise_And7/1
  Bitwise_And7/1 -> tws_7/1, AndN/7, Scope/7
  BS_Req/8 -> cmp_8/1, Scope8/1  "<testSig_EISGov_PWinNegLo>"
  BS_Result/8 -> cmp_8/2, Scope8/2  "<EISGov_PWinNegLo>"
  cmp_8/1 -> Bitwise_And8/1
  Bitwise_And8/1 -> tws_8/1, AndN/8, Scope/8
  BS_Req/9 -> cmp_9/1, Scope9/1  "<testSig_EISGov_KiCurrLo_mp>"
  BS_Result/9 -> cmp_9/2, Scope9/2  "<EISGov_KiCurrLo_mp>"
  cmp_9/1 -> Bitwise_And9/1
  Bitwise_And9/1 -> tws_9/1, AndN/9, Scope/9
  BS_Req/10 -> cmp_10/1, Scope10/1  "<testSig_EISGov_KiPosCurrLo_mp>"
  BS_Result/10 -> cmp_10/2, Scope10/2  "<EISGov_KiPosCurrLo_mp>"
  cmp_10/1 -> Bitwise_And10/1
  Bitwise_And10/1 -> tws_10/1, AndN/10, Scope/10
  BS_Req/11 -> cmp_11/1, Scope11/1  "<testSig_EISGov_KiNegCurrLo_mp>"
  BS_Result/11 -> cmp_11/2, Scope11/2  "<EISGov_KiNegCurrLo_mp>"
  cmp_11/1 -> Bitwise_And11/1
  Bitwise_And11/1 -> tws_11/1, AndN/11, Scope/11
  BS_Req/12 -> cmp_12/1, Scope12/1  "<testSig_EISGov_IWinPosLo>"
  BS_Result/12 -> cmp_12/2, Scope12/2  "<EISGov_IWinPosLo>"
  cmp_12/1 -> Bitwise_And12/1
  Bitwise_And12/1 -> tws_12/1, AndN/12, Scope/12
  BS_Req/13 -> cmp_13/1, Scope13/1  "<testSig_EISGov_IWinNegLo>"
  BS_Result/13 -> cmp_13/2, Scope13/2  "<EISGov_IWinNegLo>"
  cmp_13/1 -> Bitwise_And13/1
  Bitwise_And13/1 -> tws_13/1, AndN/13, Scope/13
  BS_Req/14 -> cmp_14/1, Scope14/1  "<testSig_EISGov_KpCurrHi_mp>"
  BS_Result/14 -> cmp_14/2, Scope14/2  "<EISGov_KpCurrHi_mp>"
  cmp_14/1 -> Bitwise_And14/1
  Bitwise_And14/1 -> tws_14/1, AndN/14, Scope/14
  BS_Req/15 -> cmp_15/1, Scope15/1  "<testSig_EISGov_KpPosCurrHi_mp>"
  BS_Result/15 -> cmp_15/2, Scope15/2  "<EISGov_KpPosCurrHi_mp>"
  cmp_15/1 -> Bitwise_And15/1
  Bitwise_And15/1 -> tws_15/1, AndN/15, Scope/15
  BS_Req/16 -> cmp_16/1, Scope16/1  "<testSig_EISGov_KpNegCurrHi_mp>"
  BS_Result/16 -> cmp_16/2, Scope16/2  "<EISGov_KpNegCurrHi_mp>"
  cmp_16/1 -> Bitwise_And16/1
  Bitwise_And16/1 -> tws_16/1, AndN/16, Scope/16
  BS_Req/17 -> cmp_17/1, Scope17/1  "<testSig_EISGov_PWinPosHi>"
  BS_Result/17 -> cmp_17/2, Scope17/2  "<EISGov_PWinPosHi>"
  cmp_17/1 -> Bitwise_And17/1
  Bitwise_And17/1 -> tws_17/1, AndN/17, Scope/17
  BS_Req/18 -> cmp_18/1, Scope18/1  "<testSig_EISGov_PWinNegHi>"
  BS_Result/18 -> cmp_18/2, Scope18/2  "<EISGov_PWinNegHi>"
  cmp_18/1 -> Bitwise_And18/1
  Bitwise_And18/1 -> tws_18/1, AndN/18, Scope/18
  BS_Req/19 -> cmp_19/1, Scope19/1  "<testSig_EISGov_KiCurrHi_mp>"
  BS_Result/19 -> cmp_19/2, Scope19/2  "<EISGov_KiCurrHi_mp>"
  cmp_19/1 -> Bitwise_And19/1
  Bitwise_And19/1 -> tws_19/1, AndN/19, Scope/19
  BS_Req/20 -> cmp_20/1, Scope20/1  "<testSig_EISGov_KiPosCurrHi_mp>"
  BS_Result/20 -> cmp_20/2, Scope20/2  "<EISGov_KiPosCurrHi_mp>"
  cmp_20/1 -> Bitwise_And20/1
  Bitwise_And20/1 -> tws_20/1, AndN/20, Scope/20
  BS_Req/21 -> cmp_21/1, Scope21/1  "<testSig_EISGov_KiNegCurrHi_mp>"
  BS_Result/21 -> cmp_21/2, Scope21/2  "<EISGov_KiNegCurrHi_mp>"
  cmp_21/1 -> Bitwise_And21/1
  Bitwise_And21/1 -> tws_21/1, AndN/21, Scope/21
  BS_Req/22 -> cmp_22/1, Scope22/1  "<testSig_EISGov_IWinPosHi>"
  BS_Result/22 -> cmp_22/2, Scope22/2  "<EISGov_IWinPosHi>"
  cmp_22/1 -> Bitwise_And22/1
  Bitwise_And22/1 -> tws_22/1, AndN/22, Scope/22
  BS_Req/23 -> cmp_23/1, Scope23/1  "<testSig_EISGov_IWinNegHi>"
  BS_Result/23 -> cmp_23/2, Scope23/2  "<EISGov_IWinNegHi>"
  cmp_23/1 -> Bitwise_And23/1
  Bitwise_And23/1 -> tws_23/1, AndN/23, Scope/23
  BS_Req/24 -> cmp_24/1, Scope24/1  "<testSig_EISGov_trqReq>"
  BS_Result/24 -> cmp_24/2, Scope24/2  "<EISGov_trqReq>"
  cmp_24/1 -> Bitwise_And24/1
  Bitwise_And24/1 -> tws_24/1, AndN/24, Scope/24
